simulink model "master_thesis"  (R2023a)
settings: Solver=ode45  StartTime=0.0  StopTime=50  FixedStep=0.001  RelTol=1e-3
values from neighbouring files (symbols this model uses):
  beta = 0.1    [computational_time.m]    (also in final_simulation.m; init_script.m)
  beta_r = 0.5    [final_simulation.m]
  D = 0.1    [computational_time.m]    (also in dampingMatrix.m = reshape([0.0,0.0,0.0,0.0,beta,t2,0.0,t2,beta./3.0],[3,3]); final_simulation.m; init_script.m; multiple_frame_plot.m)
  g = 9.81    [computational_time.m]    (also in final_simulation.m; init_script.m)
  k = 1    [computational_time.m]    (also in final_simulation.m; init_script.m = 0.1)
  Kd = -K(2)    [final_simulation.m]
  Kp = -K(1)    [final_simulation.m]
  L = 1    [computational_time.m]    (also in coriolisMatrix.m = ct{1}; final_simulation.m; init_script.m; multiple_frame_plot.m)
  m = 1    [computational_time.m]    (also in coriolisMatrix.m = ct{2}; final_simulation.m; init_script.m)
  theta_dot_init = zeros(3, 1)    [final_simulation.m]
  theta_init = [0; pi/4; -pi/4]    [final_simulation.m]
undefined symbols (not defined in the file or in its folder): collocatedFL, DiscIntNeverNeededParam, RSoft_dynamics
settings Model: Creator=Utente  LastModifiedBy=danie
settings OptimizationCC: ReuseModelBlockBuffer=off
settings DebuggingCC: UnconnectedInputMsg=warning  UnconnectedOutputMsg=warning  UnconnectedLineMsg=warning
settings ModelReferenceCC: EnableRefExpFcnMdlSchedulingChecks=on
settings RTWCC: DLArmComputeVersion=19.05

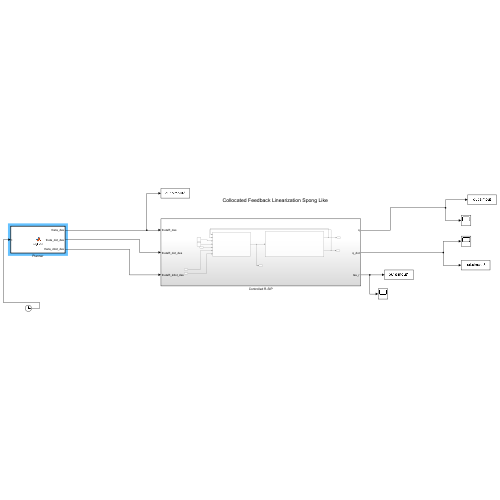
[thumbnail: Simulink's stored preview of the top-level diagram]
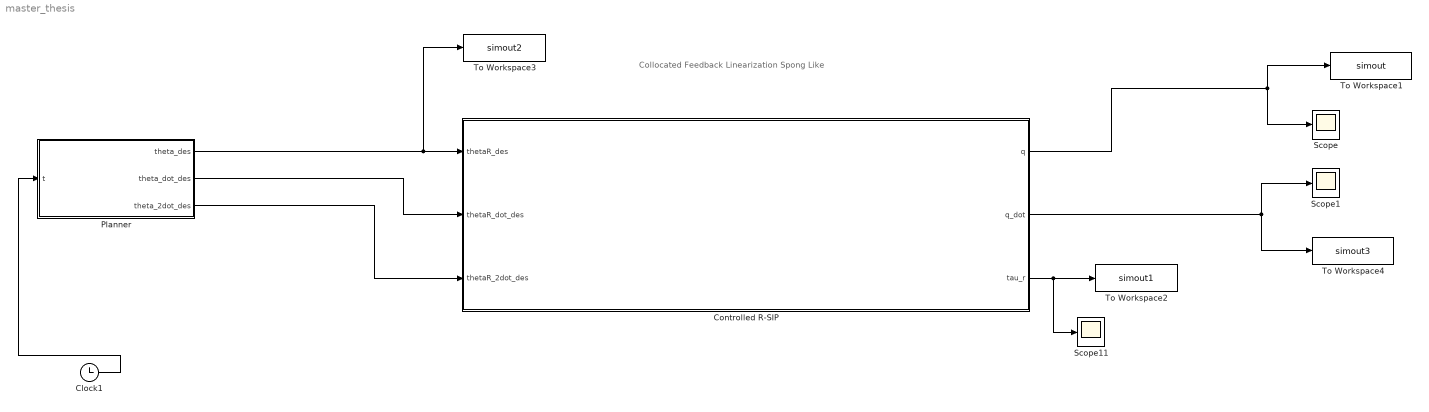
== system master_thesis ==
  note: Collocated Feedback Linearization Spong Like
  Clock1 : Clock
  Controlled R-SIP : Subsystem
  Planner : MATLAB Function  TreatAsAtomicUnit=on
  Scope : Scope
  Scope1 : Scope
  Scope11 : Scope
  To Workspace1 : ToWorkspace  VariableName=simout  SaveFormat=Timeseries  SampleTime=-1
  To Workspace2 : ToWorkspace  VariableName=simout1  SaveFormat=Timeseries  SampleTime=-1
  To Workspace3 : ToWorkspace  VariableName=simout2  SaveFormat=Timeseries  SampleTime=-1
  To Workspace4 : ToWorkspace  VariableName=simout3  SaveFormat=Timeseries  SampleTime=-1
  wires:
  Planner/1(theta_des) -> To Workspace3/1, Controlled R-SIP/1(thetaR_des)
  Clock1/1 -> Planner/1(t)
  Controlled R-SIP/1(q) -> Scope/1, To Workspace1/1
  Controlled R-SIP/2(q_dot) -> To Workspace4/1, Scope1/1
  Controlled R-SIP/3(tau_r) -> Scope11/1, To Workspace2/1
  Planner/2(theta_dot_des) -> Controlled R-SIP/2(thetaR_dot_des)
  Planner/3(theta_2dot_des) -> Controlled R-SIP/3(thetaR_2dot_des)

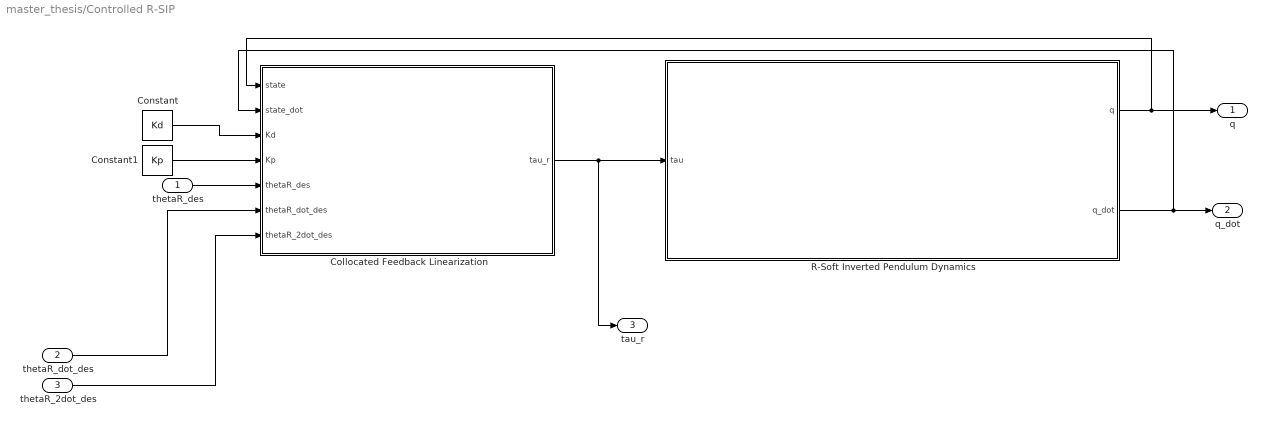
== system master_thesis/Controlled R-SIP ==
  thetaR_des : Inport
  thetaR_dot_des : Inport  Port=2
  thetaR_2dot_des : Inport  Port=3
  Collocated Feedback Linearization : Subsystem
  Constant : Constant  Value=Kd
  Constant1 : Constant  Value=Kp
  R-Soft Inverted Pendulum Dynamics : Subsystem
  q : Outport
  q_dot : Outport  Port=2
  tau_r : Outport  Port=3
  wires:
  thetaR_dot_des/1 -> Collocated Feedback Linearization/6(thetaR_dot_des)
  R-Soft Inverted Pendulum Dynamics/1(q) -> q/1, Collocated Feedback Linearization/1(state)
  thetaR_des/1 -> Collocated Feedback Linearization/5(thetaR_des)
  R-Soft Inverted Pendulum Dynamics/2(q_dot) -> q_dot/1, Collocated Feedback Linearization/2(state_dot)
  Collocated Feedback Linearization/1(tau_r) -> tau_r/1, R-Soft Inverted Pendulum Dynamics/1(tau)
  Constant/1 -> Collocated Feedback Linearization/3(Kd)
  Constant1/1 -> Collocated Feedback Linearization/4(Kp)
  thetaR_2dot_des/1 -> Collocated Feedback Linearization/7(thetaR_2dot_des)

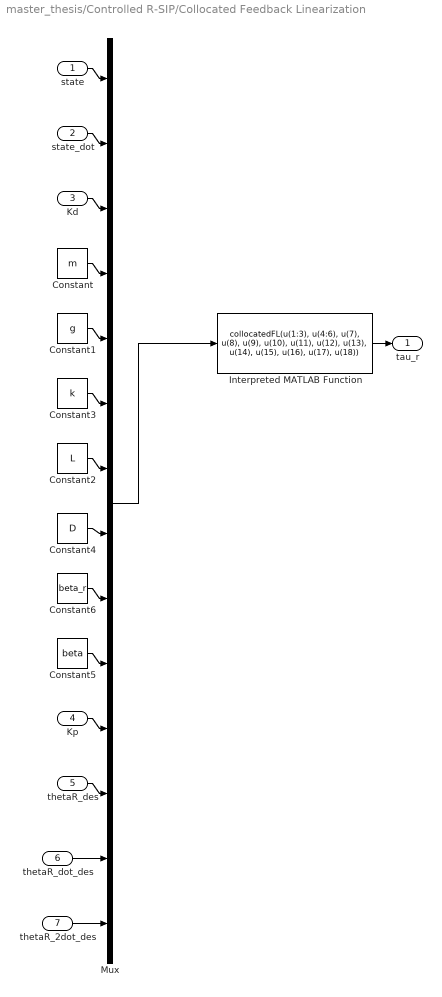
== system master_thesis/Controlled R-SIP/Collocated Feedback Linearization ==
  state : Inport
  state_dot : Inport  Port=2
  Kd : Inport  Port=3
  Kp : Inport  Port=4
  thetaR_des : Inport  Port=5
  thetaR_dot_des : Inport  Port=6
  thetaR_2dot_des : Inport  Port=7
  Constant : Constant  Value=m
  Constant1 : Constant  Value=g
  Constant2 : Constant  Value=L
  Constant3 : Constant  Value=k
  Constant4 : Constant  Value=D
  Constant5 : Constant  Value=beta
  Constant6 : Constant  Value=beta_r
  Interpreted MATLAB Function : MATLABFcn  MATLABFcn=collocatedFL(u(1:3), u(4:6), u(7), u(8), u(9), u(10), u(11), u(12), u(13), u(14), u(15), u(16), u(17), u(18))
  Mux : Mux  Inputs=14
  tau_r : Outport
  wires:
  Mux/1 -> Interpreted MATLAB Function/1
  Kd/1 -> Mux/3
  Constant2/1 -> Mux/7
  Constant1/1 -> Mux/5
  Constant/1 -> Mux/4
  Constant3/1 -> Mux/6
  Interpreted MATLAB Function/1 -> tau_r/1
  state_dot/1 -> Mux/2
  Constant4/1 -> Mux/8
  state/1 -> Mux/1
  thetaR_des/1 -> Mux/12
  Kp/1 -> Mux/11
  Constant5/1 -> Mux/10
  Constant6/1 -> Mux/9
  thetaR_dot_des/1 -> Mux/13
  thetaR_2dot_des/1 -> Mux/14

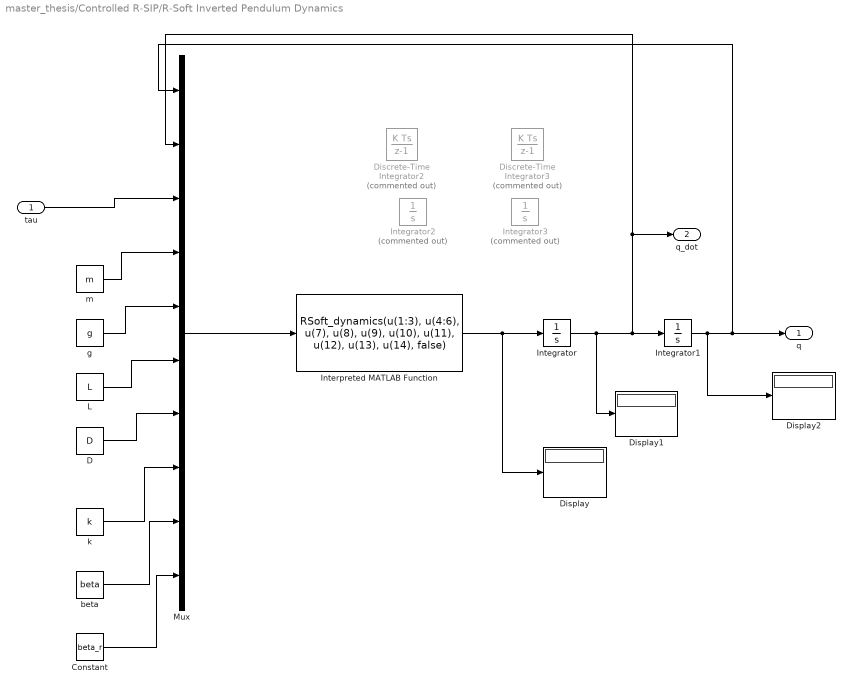
== system master_thesis/Controlled R-SIP/R-Soft Inverted Pendulum Dynamics ==
  tau : Inport
  Constant : Constant  Value=beta_r
  D : Constant  Value=D
  Discrete-Time Integrator2 : DiscreteIntegrator  Commented=on  InitialCondition=theta_dot_init  SampleTime=-1  ICPrevOutput=DiscIntNeverNeededParam  ICPrevScaledInput=DiscIntNeverNeededParam
  Discrete-Time Integrator3 : DiscreteIntegrator  Commented=on  InitialCondition=theta_init  SampleTime=-1  ICPrevOutput=DiscIntNeverNeededParam  ICPrevScaledInput=DiscIntNeverNeededParam
  Display : Display
  Display1 : Display
  Display2 : Display
  Integrator : Integrator  InitialCondition=theta_dot_init
  Integrator1 : Integrator  InitialCondition=theta_init
  Integrator2 : Integrator  Commented=on  InitialCondition=theta_dot_init
  Integrator3 : Integrator  Commented=on  InitialCondition=theta_init
  Interpreted MATLAB Function : MATLABFcn  MATLABFcn=RSoft_dynamics(u(1:3), u(4:6), u(7), u(8), u(9), u(10), u(11), u(12), u(13), u(14), false)
  L : Constant  Value=L
  Mux : Mux  Inputs=10
  beta : Constant  Value=beta
  g : Constant  Value=g
  k : Constant  Value=k
  m : Constant  Value=m
  q : Outport
  q_dot : Outport  Port=2
  wires:
  Integrator1/1 -> Display2/1, q/1, Mux/1
  g/1 -> Mux/5
  beta/1 -> Mux/9
  k/1 -> Mux/8
  m/1 -> Mux/4
  tau/1 -> Mux/3
  Integrator/1 -> Display1/1, Integrator1/1, q_dot/1, Mux/2
  L/1 -> Mux/6
  D/1 -> Mux/7
  Mux/1 -> Interpreted MATLAB Function/1
  Interpreted MATLAB Function/1 -> Integrator/1, Display/1
  Constant/1 -> Mux/10

== matlab function master_thesis/Planner ==
  data: t input; theta_des output; theta_dot_des output; theta_2dot_des output
function [theta_des, theta_dot_des, theta_2dot_des] = trajGen(t)
%% Arctg -pi/2 -> pi/2
% theta_des = atan(t - 15);
% theta_dot_des = 1/((t - 15)^2 + 1);
% theta_2dot_des = -(2*t - 30)/((t - 15)^2 + 1)^2;

%% Step -pi/2 -> pi/2
% if(t <= 15)
%     theta_des = -pi/2;
% else
%     theta_des = pi/2;
% end
% 
% theta_dot_des = 0;
% theta_2dot_des = 0;

%% Sin
% magnitude = pi;
% freq = 0.1;
% phase = 0.0;
% mean_value = pi/2;
% 
% % theta_des
% theta_des = mean_value + magnitude*sin((2*pi*freq)*t + phase);
% theta_dot_des = magnitude*(2*pi*freq)*cos((2*pi*freq)*t + phase);
% theta_2dot_des = -magnitude*((2*pi*freq)^2)*sin((2*pi*freq)*t + phase);

%% Chirp
magnitude = pi/3;
freq = 0.01;
phase = 0.0;
mean_value = pi/2;

% theta_des
theta_des = mean_value + magnitude*sin((2*pi*freq)*t^2 + phase);
theta_dot_des = (2*t)*magnitude*(2*pi*freq)*cos((2*pi*freq)*t^2 + phase);
theta_2dot_des = -(4*t^2)*magnitude*((2*pi*freq)^2)*sin((2*pi*freq)*t^2 + phase);
end
